simulink model "lab5_monocontur"  (R2023b)
settings: Solver=ode45  StartTime=0.0  StopTime=400  RelTol=1e-3
settings Model: Creator=Daniela  LastModifiedBy=Daniela

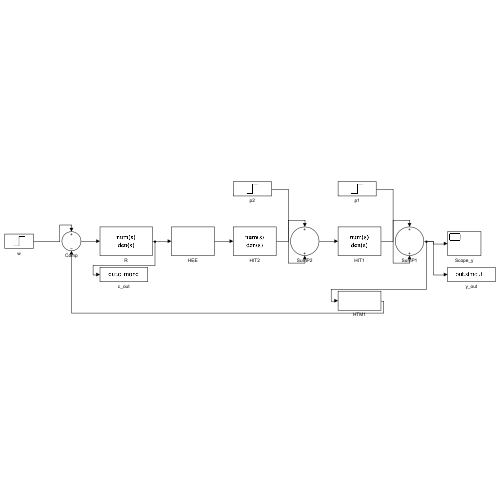
[thumbnail: Simulink's stored preview of the top-level diagram]
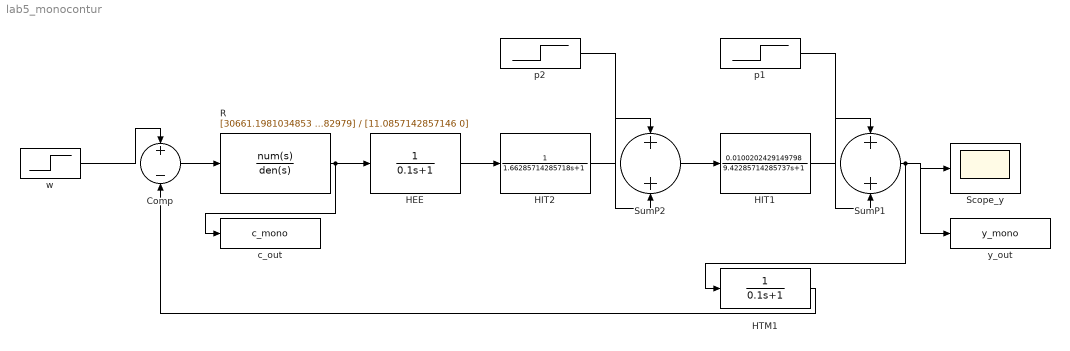
== system lab5_monocontur ==
  Comp : Sum  Inputs=+-
  HEE : TransferFcn  Numerator=1  Denominator=[0.1 1]
  HIT1 : TransferFcn  Numerator=0.0100202429149798  Denominator=[9.42285714285737 1]
  HIT2 : TransferFcn  Numerator=1  Denominator=[1.66285714285718 1]
  HTM1 : TransferFcn  Numerator=1  Denominator=[0.1 1]
  R : TransferFcn  Numerator=[30661.1981034853 2765.82972582979]  Denominator=[11.0857142857146 0]
  Scope_y : Scope
  SumP1 : Sum
  SumP2 : Sum
  c_out : ToWorkspace  VariableName=c_mono  SampleTime=-1
  p1 : Step  Time=0  After=0  SampleTime=0
  p2 : Step  Time=80  SampleTime=0
  w : Step  Time=0  After=0.1  SampleTime=0
  y_out : ToWorkspace  VariableName=y_mono  SampleTime=-1
  wires:
  w/1 -> Comp/1
  Comp/1 -> R/1
  R/1 -> HEE/1, c_out/1
  HEE/1 -> HIT2/1
  HIT2/1 -> SumP2/1
  p2/1 -> SumP2/2
  SumP2/1 -> HIT1/1
  HIT1/1 -> SumP1/1
  p1/1 -> SumP1/2
  SumP1/1 -> Scope_y/1, y_out/1, HTM1/1
  HTM1/1 -> Comp/2
